simulink library "dyn"  (Simulink 8.2)
settings: Solver=ode45  StartTime=0.0  StopTime=10.0  RelTol=1e-3
undefined symbols (not defined in the file or in its folder): KVSE_AccelWeightOffset_rat, KVSE_AccelWeightSlope_rat, KVSE_StartModeInDelaySpd_kph, KVSE_StartModeInWheelSpd_kph, KVSE_StartModeOutWheelSpd_kph, KVSE_TurnModeInYawRate_degps, KVSE_TurnModeOutYawRate_degps, KVSE_WheelSpdAdjust_rat, KVSE_WheelWeightOffset_rat, KVSE_WheelWeightSlope_rat
libraries: simulink x6
(part 1 of 2)
settings Model: RequirementInfo="{}  %GIDa_9c3e9883_6bb3_4e31_949e_ba791919a9a8"  Creator=16027  LastModifiedBy=14014  CovModelRefEnable=off

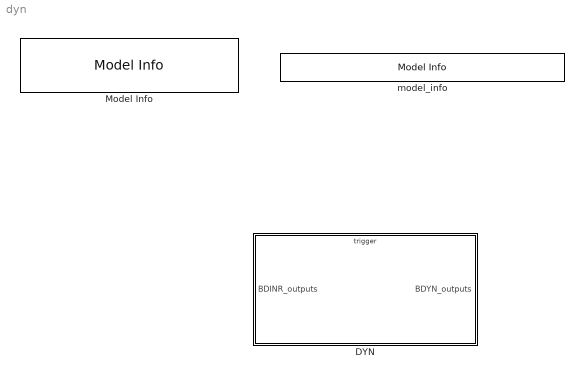
== system dyn ==
  DYN : Subsystem
  Model Info : simulink/Model-Wide Utilities/Model Info  InitialBlockCM=None  BlockCM=none  Frame=on  DisplayStringWithTags=|  HorizontalTextAlignment=Left  LeftAlignmentValue=0.02  SourceBlockDiagram=dyn  TagMaxNumber=20
      | Model Version        : %<ModelVersion>
      | Creator                   : %<Creator>
      | Last Modified by    : %<LastModifiedBy>
  model_info : simulink/Model-Wide Utilities/Model Info  InitialBlockCM=None  BlockCM=None  Frame=on  DisplayStringWithTags=$Id: dyn.mdl 1524 2016-11-04 02:29:39Z chimotsai $  HorizontalTextAlignment=Center  LeftAlignmentValue=0.5  SourceBlockDiagram=dyn  TagMaxNumber=20

== system dyn/DYN ==
  BDINR_outputs : Inport  OutDataTypeStr=Bus: BDINR_outputs
  trig_DYN : TriggerPort  TriggerType=function-call  PortDimensions=1
  Bus Creator : BusCreator  Inputs=1  OutDataTypeStr=Bus: BDYN_outputs
  Bus Selector1 : BusSelector  OutputSignals=VDINR_RRWheelSpeed_kph,VDINR_LRWheelSpeed_kph,VDINR_RFWheelSpeed_kph,VDINR_LFWheelSpeed_kph,VDINR_LongAccel_G,VDINR_YawRate_degps
  Vehicle Speed Estimation : Subsystem  RequirementInfo={} %GIDa_6aef2b2b_4aef_4102_9e64_605181178381
  BDYN_outputs : Outport  OutDataTypeStr=Bus: BDYN_outputs
  wires:
  Bus Selector1/1 -> Vehicle Speed Estimation/1(VDINR_RRWheelSpeed_kph)  "<VDINR_RRWheelSpeed_kph>"
  Vehicle Speed Estimation/1(VVSE_VehSpdEst_kph) -> Bus Creator/1
  BDINR_outputs/1 -> Bus Selector1/1
  Bus Creator/1 -> BDYN_outputs/1  "BDYN_outputs"
  Bus Selector1/2 -> Vehicle Speed Estimation/2(VDINR_LRWheelSpeed_kph)  "<VDINR_LRWheelSpeed_kph>"
  Bus Selector1/3 -> Vehicle Speed Estimation/3(VDINR_RFWheelSpeed_kph)  "<VDINR_RFWheelSpeed_kph>"
  Bus Selector1/4 -> Vehicle Speed Estimation/4(VDINR_LFWheelSpeed_kph)  "<VDINR_LFWheelSpeed_kph>"
  Bus Selector1/5 -> Vehicle Speed Estimation/5(VDINR_LongAccel_G)  "<VDINR_LongAccel_G>"
  Bus Selector1/6 -> Vehicle Speed Estimation/6(VDINR_YawRate_degps)  "<VDINR_YawRate_degps>"

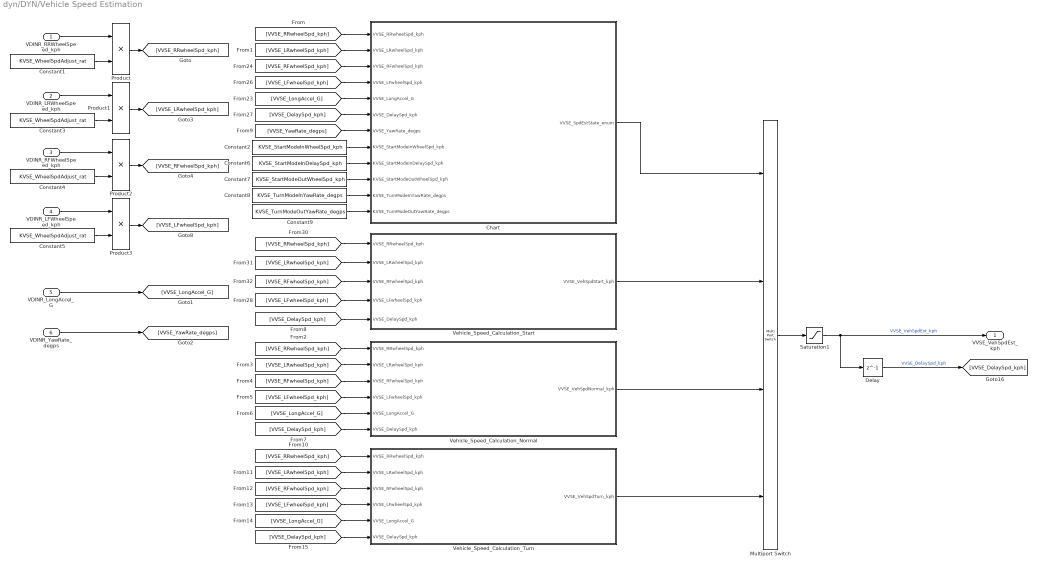
== system dyn/DYN/Vehicle Speed Estimation ==
  VDINR_RRWheelSpeed_kph : Inport
  VDINR_LRWheelSpeed_kph : Inport  Port=2
  VDINR_RFWheelSpeed_kph : Inport  Port=3
  VDINR_LFWheelSpeed_kph : Inport  Port=4
  VDINR_LongAccel_G : Inport  Port=5
  VDINR_YawRate_degps : Inport  Port=6
  Chart : Stateflow chart  TreatAsAtomicUnit=on
  Constant{1,3..5} (4 alike) : Constant  Value=KVSE_WheelSpdAdjust_rat
  Constant2 : Constant  Value=KVSE_StartModeInWheelSpd_kph
  Constant6 : Constant  Value=KVSE_StartModeInDelaySpd_kph
  Constant7 : Constant  Value=KVSE_StartModeOutWheelSpd_kph
  Constant8 : Constant  Value=KVSE_TurnModeInYawRate_degps
  Constant9 : Constant  Value=KVSE_TurnModeOutYawRate_degps
  Delay : Delay  DelayLength=1  InitialCondition=0
  Multiport Switch : MultiPortSwitch
  Product{,1..3} (4 alike) : Product
  Saturation1 : Saturate  UpperLimit=220  LowerLimit=0
  "Vehicle_Speed_Calculation_Normal " : Subsystem
  Vehicle_Speed_Calculation_Start : Subsystem
  "Vehicle_Speed_Calculation_Turn " : Subsystem
  VVSE_VehSpdEst_kph : Outport
  wires:
  Delay/1 -> [VVSE_DelaySpd_kph]  "VVSE_DelaySpd_kph"
  Saturation1/1 -> VVSE_VehSpdEst_kph/1, Delay/1  "VVSE_VehSpdEst_kph"
  [VVSE_LRwheelSpd_kph] -> "Vehicle_Speed_Calculation_Normal "/2(VVSE_LRwheelSpd_kph)
  [VVSE_RFwheelSpd_kph] -> "Vehicle_Speed_Calculation_Normal "/3(VVSE_RFwheelSpd_kph)
  [VVSE_LFwheelSpd_kph] -> "Vehicle_Speed_Calculation_Normal "/4(VVSE_LFwheelSpd_kph)
  [VVSE_LongAccel_G] -> "Vehicle_Speed_Calculation_Normal "/5(VVSE_LongAccel_G)
  [VVSE_DelaySpd_kph] -> "Vehicle_Speed_Calculation_Normal "/6(VVSE_DelaySpd_kph)
  [VVSE_RRwheelSpd_kph] -> Chart/1(VVSE_RRwheelSpd_kph)
  [VVSE_LRwheelSpd_kph] -> Chart/2(VVSE_LRwheelSpd_kph)
  [VVSE_LFwheelSpd_kph] -> Chart/4(VVSE_LFwheelSpd_kph)
  [VVSE_RFwheelSpd_kph] -> Chart/3(VVSE_RFwheelSpd_kph)
  [VVSE_DelaySpd_kph] -> Chart/6(VVSE_DelaySpd_kph)
  [VVSE_LongAccel_G] -> Chart/5(VVSE_LongAccel_G)
  Multiport Switch/1 -> Saturation1/1
  [VVSE_RRwheelSpd_kph] -> "Vehicle_Speed_Calculation_Normal "/1(VVSE_RRwheelSpd_kph)
  [VVSE_LFwheelSpd_kph] -> Vehicle_Speed_Calculation_Start/4(VVSE_LFwheelSpd_kph)
  [VVSE_RFwheelSpd_kph] -> Vehicle_Speed_Calculation_Start/3(VVSE_RFwheelSpd_kph)
  [VVSE_LRwheelSpd_kph] -> Vehicle_Speed_Calculation_Start/2(VVSE_LRwheelSpd_kph)
  [VVSE_RRwheelSpd_kph] -> Vehicle_Speed_Calculation_Start/1(VVSE_RRwheelSpd_kph)
  [VVSE_DelaySpd_kph] -> Vehicle_Speed_Calculation_Start/5(VVSE_DelaySpd_kph)
  Product/1 -> [VVSE_RRwheelSpd_kph]
  VDINR_RRWheelSpeed_kph/1 -> Product/1
  Constant1/1 -> Product/2
  Product1/1 -> [VVSE_LRwheelSpd_kph]
  VDINR_LRWheelSpeed_kph/1 -> Product1/1
  Constant3/1 -> Product1/2
  Product2/1 -> [VVSE_RFwheelSpd_kph]
  VDINR_RFWheelSpeed_kph/1 -> Product2/1
  Constant4/1 -> Product2/2
  Product3/1 -> [VVSE_LFwheelSpd_kph]
  VDINR_LFWheelSpeed_kph/1 -> Product3/1
  Constant5/1 -> Product3/2
  VDINR_LongAccel_G/1 -> [VVSE_LongAccel_G]
  "Vehicle_Speed_Calculation_Normal "/1(VVSE_VehSpdNormal_kph) -> Multiport Switch/3
  Vehicle_Speed_Calculation_Start/1(VVSE_VehSpdStart_kph) -> Multiport Switch/2
  VDINR_YawRate_degps/1 -> [VVSE_YawRate_degps]
  [VVSE_YawRate_degps] -> Chart/7(VVSE_YawRate_degps)
  Chart/1(VVSE_SpdEstState_enum) -> Multiport Switch/1
  "Vehicle_Speed_Calculation_Turn "/1(VVSE_VehSpdTurn_kph) -> Multiport Switch/4
  [VVSE_RRwheelSpd_kph] -> "Vehicle_Speed_Calculation_Turn "/1(VVSE_RRwheelSpd_kph)
  [VVSE_LRwheelSpd_kph] -> "Vehicle_Speed_Calculation_Turn "/2(VVSE_LRwheelSpd_kph)
  [VVSE_RFwheelSpd_kph] -> "Vehicle_Speed_Calculation_Turn "/3(VVSE_RFwheelSpd_kph)
  [VVSE_LFwheelSpd_kph] -> "Vehicle_Speed_Calculation_Turn "/4(VVSE_LFwheelSpd_kph)
  [VVSE_LongAccel_G] -> "Vehicle_Speed_Calculation_Turn "/5(VVSE_LongAccel_G)
  [VVSE_DelaySpd_kph] -> "Vehicle_Speed_Calculation_Turn "/6(VVSE_DelaySpd_kph)
  Constant2/1 -> Chart/8(KVSE_StartModeInWheelSpd_kph)
  Constant6/1 -> Chart/9(KVSE_StartModeInDelaySpd_kph)
  Constant7/1 -> Chart/10(KVSE_StartModeOutWheelSpd_kph)
  Constant8/1 -> Chart/11(KVSE_TurnModeInYawRate_degps)
  Constant9/1 -> Chart/12(KVSE_TurnModeOutYawRate_degps)

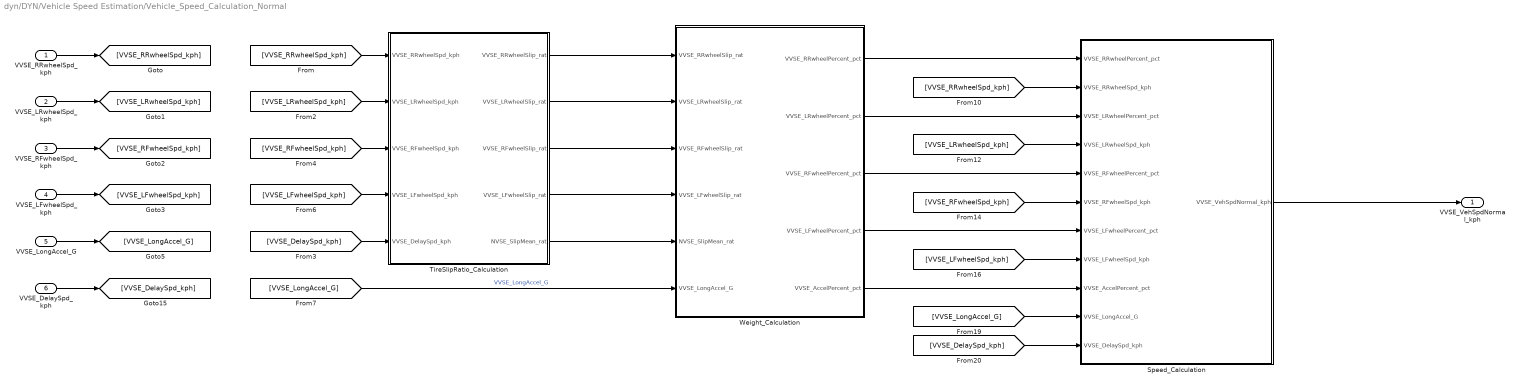
== system dyn/DYN/Vehicle Speed Estimation/Vehicle_Speed_Calculation_Normal  ==
  VVSE_RRwheelSpd_kph : Inport
  VVSE_LRwheelSpd_kph : Inport  Port=2
  VVSE_RFwheelSpd_kph : Inport  Port=3
  VVSE_LFwheelSpd_kph : Inport  Port=4
  VVSE_LongAccel_G : Inport  Port=5
  VVSE_DelaySpd_kph : Inport  Port=6
  Speed_Calculation : Subsystem
  TireSlipRatio_Calculation : Subsystem
  Weight_Calculation : Subsystem  RequirementInfo={} %GIDa_581bf922_3c60_4f28_b9a5_a6cc319ffbb8
  VVSE_VehSpdNormal_kph : Outport
  wires:
  [VVSE_RRwheelSpd_kph] -> TireSlipRatio_Calculation/1(VVSE_RRwheelSpd_kph)
  [VVSE_LongAccel_G] -> Weight_Calculation/6(VVSE_LongAccel_G)  "VVSE_LongAccel_G"
  Speed_Calculation/1(VVSE_VehSpdNormal_kph) -> VVSE_VehSpdNormal_kph/1
  VVSE_LongAccel_G/1 -> [VVSE_LongAccel_G]
  VVSE_DelaySpd_kph/1 -> [VVSE_DelaySpd_kph]
  Weight_Calculation/5(VVSE_AccelPercent_pct) -> Speed_Calculation/9(VVSE_AccelPercent_pct)
  [VVSE_LongAccel_G] -> Speed_Calculation/10(VVSE_LongAccel_G)
  [VVSE_DelaySpd_kph] -> Speed_Calculation/11(VVSE_DelaySpd_kph)
  Weight_Calculation/2(VVSE_LRwheelPercent_pct) -> Speed_Calculation/3(VVSE_LRwheelPercent_pct)
  [VVSE_RRwheelSpd_kph] -> Speed_Calculation/2(VVSE_RRwheelSpd_kph)
  Weight_Calculation/1(VVSE_RRwheelPercent_pct) -> Speed_Calculation/1(VVSE_RRwheelPercent_pct)
  [VVSE_LRwheelSpd_kph] -> Speed_Calculation/4(VVSE_LRwheelSpd_kph)
  Weight_Calculation/3(VVSE_RFwheelPercent_pct) -> Speed_Calculation/5(VVSE_RFwheelPercent_pct)
  [VVSE_RFwheelSpd_kph] -> Speed_Calculation/6(VVSE_RFwheelSpd_kph)
  Weight_Calculation/4(VVSE_LFwheelPercent_pct) -> Speed_Calculation/7(VVSE_LFwheelPercent_pct)
  VVSE_LRwheelSpd_kph/1 -> [VVSE_LRwheelSpd_kph]
  VVSE_RFwheelSpd_kph/1 -> [VVSE_RFwheelSpd_kph]
  VVSE_LFwheelSpd_kph/1 -> [VVSE_LFwheelSpd_kph]
  VVSE_RRwheelSpd_kph/1 -> [VVSE_RRwheelSpd_kph]
  [VVSE_LRwheelSpd_kph] -> TireSlipRatio_Calculation/2(VVSE_LRwheelSpd_kph)
  [VVSE_RFwheelSpd_kph] -> TireSlipRatio_Calculation/3(VVSE_RFwheelSpd_kph)
  [VVSE_LFwheelSpd_kph] -> TireSlipRatio_Calculation/4(VVSE_LFwheelSpd_kph)
  [VVSE_DelaySpd_kph] -> TireSlipRatio_Calculation/5(VVSE_DelaySpd_kph)
  TireSlipRatio_Calculation/5(NVSE_SlipMean_rat) -> Weight_Calculation/5(NVSE_SlipMean_rat)
  TireSlipRatio_Calculation/4(VVSE_LFwheelSlip_rat) -> Weight_Calculation/4(VVSE_LFwheelSlip_rat)
  TireSlipRatio_Calculation/3(VVSE_RFwheelSlip_rat) -> Weight_Calculation/3(VVSE_RFwheelSlip_rat)
  TireSlipRatio_Calculation/2(VVSE_LRwheelSlip_rat) -> Weight_Calculation/2(VVSE_LRwheelSlip_rat)
  TireSlipRatio_Calculation/1(VVSE_RRwheelSlip_rat) -> Weight_Calculation/1(VVSE_RRwheelSlip_rat)
  [VVSE_LFwheelSpd_kph] -> Speed_Calculation/8(VVSE_LFwheelSpd_kph)

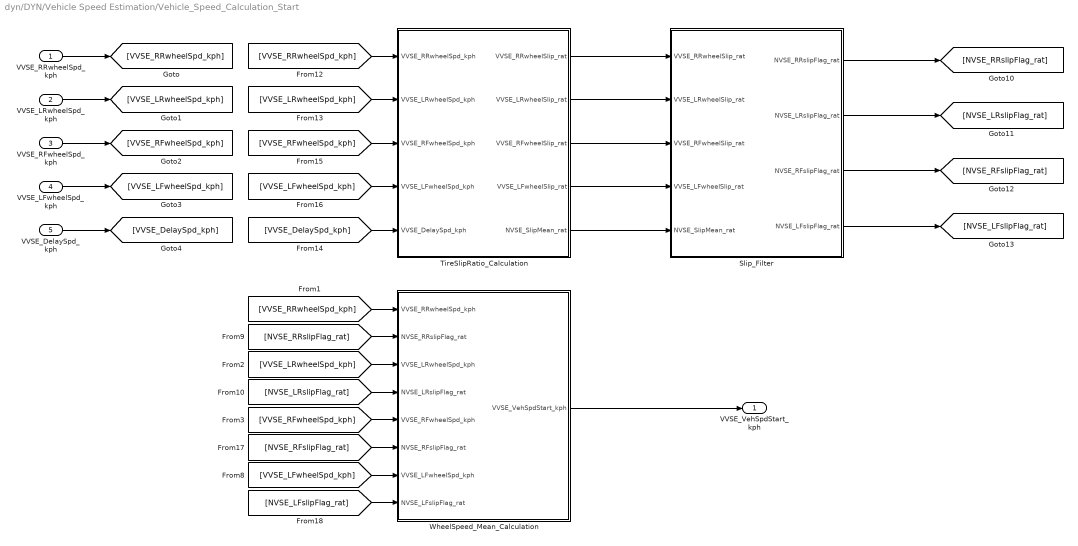
== system dyn/DYN/Vehicle Speed Estimation/Vehicle_Speed_Calculation_Start ==
  VVSE_RRwheelSpd_kph : Inport
  VVSE_LRwheelSpd_kph : Inport  Port=2
  VVSE_RFwheelSpd_kph : Inport  Port=3
  VVSE_LFwheelSpd_kph : Inport  Port=4
  VVSE_DelaySpd_kph : Inport  Port=5
  Slip_Filter : Subsystem
  TireSlipRatio_Calculation : Subsystem  RequirementInfo={} %GIDa_4f43d894_ac8b_41fb_96be_b9fe366c055a
  WheelSpeed_Mean_Calculation : Subsystem
  VVSE_VehSpdStart_kph : Outport
  wires:
  VVSE_LRwheelSpd_kph/1 -> [VVSE_LRwheelSpd_kph]
  VVSE_RFwheelSpd_kph/1 -> [VVSE_RFwheelSpd_kph]
  VVSE_LFwheelSpd_kph/1 -> [VVSE_LFwheelSpd_kph]
  VVSE_RRwheelSpd_kph/1 -> [VVSE_RRwheelSpd_kph]
  [VVSE_RRwheelSpd_kph] -> TireSlipRatio_Calculation/1(VVSE_RRwheelSpd_kph)
  [VVSE_LRwheelSpd_kph] -> TireSlipRatio_Calculation/2(VVSE_LRwheelSpd_kph)
  [VVSE_DelaySpd_kph] -> TireSlipRatio_Calculation/5(VVSE_DelaySpd_kph)
  [VVSE_LFwheelSpd_kph] -> TireSlipRatio_Calculation/4(VVSE_LFwheelSpd_kph)
  [VVSE_RFwheelSpd_kph] -> TireSlipRatio_Calculation/3(VVSE_RFwheelSpd_kph)
  VVSE_DelaySpd_kph/1 -> [VVSE_DelaySpd_kph]
  Slip_Filter/1(NVSE_RRslipFlag_rat) -> [NVSE_RRslipFlag_rat]
  Slip_Filter/2(NVSE_LRslipFlag_rat) -> [NVSE_LRslipFlag_rat]
  Slip_Filter/3(NVSE_RFslipFlag_rat) -> [NVSE_RFslipFlag_rat]
  Slip_Filter/4(NVSE_LFslipFlag_rat) -> [NVSE_LFslipFlag_rat]
  [VVSE_RRwheelSpd_kph] -> WheelSpeed_Mean_Calculation/1(VVSE_RRwheelSpd_kph)
  [NVSE_RRslipFlag_rat] -> WheelSpeed_Mean_Calculation/2(NVSE_RRslipFlag_rat)
  [VVSE_LRwheelSpd_kph] -> WheelSpeed_Mean_Calculation/3(VVSE_LRwheelSpd_kph)
  [NVSE_LRslipFlag_rat] -> WheelSpeed_Mean_Calculation/4(NVSE_LRslipFlag_rat)
  [VVSE_RFwheelSpd_kph] -> WheelSpeed_Mean_Calculation/5(VVSE_RFwheelSpd_kph)
  [NVSE_RFslipFlag_rat] -> WheelSpeed_Mean_Calculation/6(NVSE_RFslipFlag_rat)
  [VVSE_LFwheelSpd_kph] -> WheelSpeed_Mean_Calculation/7(VVSE_LFwheelSpd_kph)
  [NVSE_LFslipFlag_rat] -> WheelSpeed_Mean_Calculation/8(NVSE_LFslipFlag_rat)
  WheelSpeed_Mean_Calculation/1(VVSE_VehSpdStart_kph) -> VVSE_VehSpdStart_kph/1
  TireSlipRatio_Calculation/1(VVSE_RRwheelSlip_rat) -> Slip_Filter/1(VVSE_RRwheelSlip_rat)
  TireSlipRatio_Calculation/2(VVSE_LRwheelSlip_rat) -> Slip_Filter/2(VVSE_LRwheelSlip_rat)
  TireSlipRatio_Calculation/3(VVSE_RFwheelSlip_rat) -> Slip_Filter/3(VVSE_RFwheelSlip_rat)
  TireSlipRatio_Calculation/4(VVSE_LFwheelSlip_rat) -> Slip_Filter/4(VVSE_LFwheelSlip_rat)
  TireSlipRatio_Calculation/5(NVSE_SlipMean_rat) -> Slip_Filter/5(NVSE_SlipMean_rat)

== system dyn/DYN/Vehicle Speed Estimation/Vehicle_Speed_Calculation_Turn  ==
  VVSE_RRwheelSpd_kph : Inport
  VVSE_LRwheelSpd_kph : Inport  Port=2
  VVSE_RFwheelSpd_kph : Inport  Port=3
  VVSE_LFwheelSpd_kph : Inport  Port=4
  VVSE_LongAccel_G : Inport  Port=5
  VVSE_DelaySpd_kph : Inport  Port=6
  Speed_Calculation1 : Subsystem
  TireSlipRatio_Calculation1 : Subsystem  AncestorBlock=VSE/VSE/Vehicle Speed Estimation/Vehicle_Speed_Calculation_Normal /TireSlipRatio_Calculation
  Weight_Calculation : Subsystem
  VVSE_VehSpdTurn_kph : Outport
  wires:
  [VVSE_RRwheelSpd_kph] -> TireSlipRatio_Calculation1/1(VVSE_RRwheelSpd_kph)
  [VVSE_LongAccel_G] -> Weight_Calculation/6(VVSE_LongAccel_G)  "VVSE_LongAccel_G"
  Speed_Calculation1/1(VVSE_VehSpdTurn_kph) -> VVSE_VehSpdTurn_kph/1
  VVSE_LongAccel_G/1 -> [VVSE_LongAccel_G]
  VVSE_DelaySpd_kph/1 -> [VVSE_DelaySpd_kph]
  Weight_Calculation/5(VVSE_AccelPercent_pct) -> Speed_Calculation1/9(VVSE_AccelPercent_pct)
  [VVSE_LongAccel_G] -> Speed_Calculation1/10(VVSE_LongAccel_G)
  [VVSE_DelaySpd_kph] -> Speed_Calculation1/11(VVSE_DelaySpd_kph)
  Weight_Calculation/2(VVSE_LRwheelPercent_pct) -> Speed_Calculation1/3(VVSE_LRwheelPercent_pct)
  [VVSE_RRwheelSpd_kph] -> Speed_Calculation1/2(VVSE_RRwheelSpd_kph)
  Weight_Calculation/1(VVSE_RRwheelPercent_pct) -> Speed_Calculation1/1(VVSE_RRwheelPercent_pct)
  [VVSE_LRwheelSpd_kph] -> Speed_Calculation1/4(VVSE_LRwheelSpd_kph)
  Weight_Calculation/3(VVSE_RFwheelPercent_pct) -> Speed_Calculation1/5(VVSE_RFwheelPercent_pct)
  [VVSE_RFwheelSpd_kph] -> Speed_Calculation1/6(VVSE_RFwheelSpd_kph)
  Weight_Calculation/4(VVSE_LFwheelPercent_pct) -> Speed_Calculation1/7(VVSE_LFwheelPercent_pct)
  VVSE_LRwheelSpd_kph/1 -> [VVSE_LRwheelSpd_kph]
  VVSE_RFwheelSpd_kph/1 -> [VVSE_RFwheelSpd_kph]
  VVSE_LFwheelSpd_kph/1 -> [VVSE_LFwheelSpd_kph]
  VVSE_RRwheelSpd_kph/1 -> [VVSE_RRwheelSpd_kph]
  [VVSE_LRwheelSpd_kph] -> TireSlipRatio_Calculation1/2(VVSE_LRwheelSpd_kph)
  [VVSE_RFwheelSpd_kph] -> TireSlipRatio_Calculation1/3(VVSE_RFwheelSpd_kph)
  [VVSE_LFwheelSpd_kph] -> TireSlipRatio_Calculation1/4(VVSE_LFwheelSpd_kph)
  TireSlipRatio_Calculation1/5(NVSE_SlipMean_rat) -> Weight_Calculation/5(NVSE_SlipMean_rat)
  TireSlipRatio_Calculation1/4(VVSE_LFwheelSlip_rat) -> Weight_Calculation/4(VVSE_LFwheelSlip_rat)
  TireSlipRatio_Calculation1/3(VVSE_RFwheelSlip_rat) -> Weight_Calculation/3(VVSE_RFwheelSlip_rat)
  TireSlipRatio_Calculation1/2(VVSE_LRwheelSlip_rat) -> Weight_Calculation/2(VVSE_LRwheelSlip_rat)
  TireSlipRatio_Calculation1/1(VVSE_RRwheelSlip_rat) -> Weight_Calculation/1(VVSE_RRwheelSlip_rat)
  [VVSE_LFwheelSpd_kph] -> Speed_Calculation1/8(VVSE_LFwheelSpd_kph)

== system dyn/DYN/Vehicle Speed Estimation/Vehicle_Speed_Calculation_Normal /Speed_Calculation ==
  VVSE_RRwheelPercent_pct : Inport
  VVSE_RRwheelSpd_kph : Inport  Port=2
  VVSE_LRwheelPercent_pct : Inport  Port=3
  VVSE_LRwheelSpd_kph : Inport  Port=4
  VVSE_RFwheelPercent_pct : Inport  Port=5
  VVSE_RFwheelSpd_kph : Inport  Port=6
  VVSE_LFwheelPercent_pct : Inport  Port=7
  VVSE_LFwheelSpd_kph : Inport  Port=8
  VVSE_AccelPercent_pct : Inport  Port=9
  VVSE_LongAccel_G : Inport  Port=10
  VVSE_DelaySpd_kph : Inport  Port=11
  Add : Sum
  Add1 : Sum  Inputs=+++++
  Gain : Gain  Gain=9.81
  Gain1 : Gain  Gain=0.01
  Gain2 : Gain  Gain=3.6
  Product{,1..4} (5 alike) : Product
  VVSE_VehSpdNormal_kph : Outport
  wires:
  Gain/1 -> Gain1/1
  Product4/1 -> Add1/5
  Product/1 -> Add1/1
  Add/1 -> Product4/2
  Product1/1 -> Add1/2
  Product2/1 -> Add1/3
  Gain2/1 -> Add/1
  Product3/1 -> Add1/4
  Gain1/1 -> Gain2/1
  VVSE_RRwheelPercent_pct/1 -> Product/1
  VVSE_RFwheelPercent_pct/1 -> Product2/1
  VVSE_LongAccel_G/1 -> Gain/1
  VVSE_DelaySpd_kph/1 -> Add/2
  VVSE_LRwheelPercent_pct/1 -> Product1/1
  VVSE_LRwheelSpd_kph/1 -> Product1/2
  VVSE_AccelPercent_pct/1 -> Product4/1
  VVSE_LFwheelSpd_kph/1 -> Product3/2
  VVSE_RRwheelSpd_kph/1 -> Product/2
  VVSE_RFwheelSpd_kph/1 -> Product2/2
  VVSE_LFwheelPercent_pct/1 -> Product3/1
  Add1/1 -> VVSE_VehSpdNormal_kph/1  "VVSE_VehSpdNormal_kph"

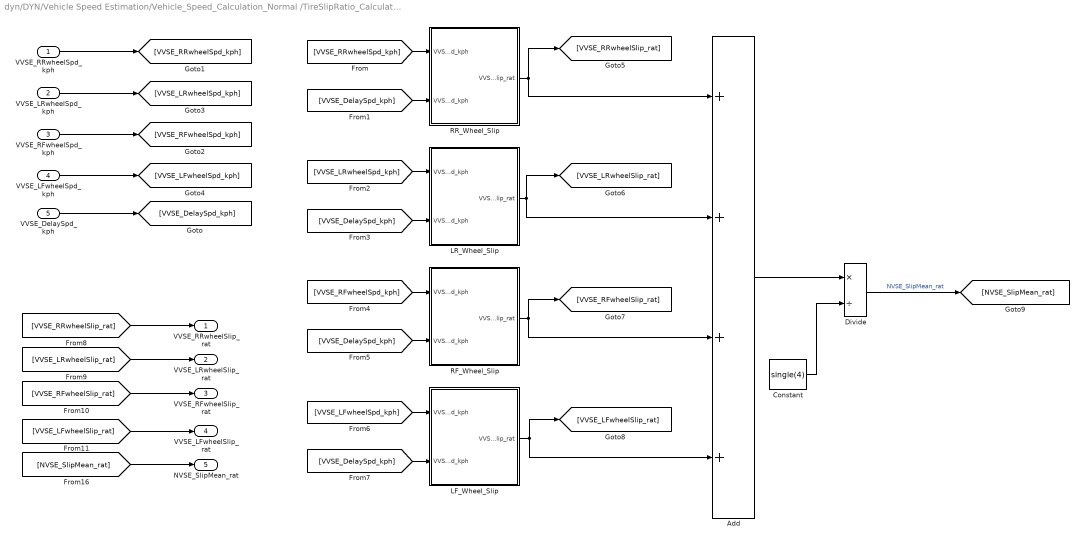
== system dyn/DYN/Vehicle Speed Estimation/Vehicle_Speed_Calculation_Normal /TireSlipRatio_Calculation ==
  VVSE_RRwheelSpd_kph : Inport
  VVSE_LRwheelSpd_kph : Inport  Port=2
  VVSE_RFwheelSpd_kph : Inport  Port=3
  VVSE_LFwheelSpd_kph : Inport  Port=4
  VVSE_DelaySpd_kph : Inport  Port=5
  Add : Sum  Inputs=++++
  Constant : Constant  Value=single(4)
  Divide : Product  Inputs=*/
  "LF_Wheel_Slip " : Subsystem
  LR_Wheel_Slip : Subsystem
  RF_Wheel_Slip : Subsystem
  RR_Wheel_Slip : Subsystem  RequirementInfo={} %GIDa_c8b2f6a2_3d64_4d29_9794_b0dc0d6a5f58
  VVSE_RRwheelSlip_rat : Outport
  VVSE_LRwheelSlip_rat : Outport  Port=2
  VVSE_RFwheelSlip_rat : Outport  Port=3
  VVSE_LFwheelSlip_rat : Outport  Port=4
  NVSE_SlipMean_rat : Outport  Port=5
  wires:
  Constant/1 -> Divide/2
  VVSE_DelaySpd_kph/1 -> [VVSE_DelaySpd_kph]
  Divide/1 -> [NVSE_SlipMean_rat]  "NVSE_SlipMean_rat"
  Add/1 -> Divide/1
  "LF_Wheel_Slip "/1(VVSE_LFwheelSlip_rat) -> [VVSE_LFwheelSlip_rat], Add/4
  [NVSE_SlipMean_rat] -> NVSE_SlipMean_rat/1
  [VVSE_DelaySpd_kph] -> RR_Wheel_Slip/2(VVSE_DelaySpd_kph)
  [VVSE_LRwheelSlip_rat] -> VVSE_LRwheelSlip_rat/1
  [VVSE_LFwheelSlip_rat] -> VVSE_LFwheelSlip_rat/1
  VVSE_RRwheelSpd_kph/1 -> [VVSE_RRwheelSpd_kph]
  RF_Wheel_Slip/1(VVSE_RFwheelSlip_rat) -> [VVSE_RFwheelSlip_rat], Add/3
  RR_Wheel_Slip/1(VVSE_RRwheelSlip_rat) -> [VVSE_RRwheelSlip_rat], Add/1
  [VVSE_RRwheelSlip_rat] -> VVSE_RRwheelSlip_rat/1
  [VVSE_RFwheelSlip_rat] -> VVSE_RFwheelSlip_rat/1
  VVSE_RFwheelSpd_kph/1 -> [VVSE_RFwheelSpd_kph]
  LR_Wheel_Slip/1(VVSE_LRwheelSlip_rat) -> Add/2, [VVSE_LRwheelSlip_rat]
  [VVSE_RFwheelSpd_kph] -> RF_Wheel_Slip/1(VVSE_RFwheelSpd_kph)
  [VVSE_DelaySpd_kph] -> RF_Wheel_Slip/2(VVSE_DelaySpd_kph)
  [VVSE_LRwheelSpd_kph] -> LR_Wheel_Slip/1(VVSE_LRwheelSpd_kph)
  VVSE_LFwheelSpd_kph/1 -> [VVSE_LFwheelSpd_kph]
  VVSE_LRwheelSpd_kph/1 -> [VVSE_LRwheelSpd_kph]
  [VVSE_DelaySpd_kph] -> LR_Wheel_Slip/2(VVSE_DelaySpd_kph)
  [VVSE_DelaySpd_kph] -> "LF_Wheel_Slip "/2(VVSE_DelaySpd_kph)
  [VVSE_LFwheelSpd_kph] -> "LF_Wheel_Slip "/1(VVSE_LFwheelSpd_kph)
  [VVSE_RRwheelSpd_kph] -> RR_Wheel_Slip/1(VVSE_RRwheelSpd_kph)

== system dyn/DYN/Vehicle Speed Estimation/Vehicle_Speed_Calculation_Normal /Weight_Calculation ==
  VVSE_RRwheelSlip_rat : Inport
  VVSE_LRwheelSlip_rat : Inport  Port=2
  VVSE_RFwheelSlip_rat : Inport  Port=3
  VVSE_LFwheelSlip_rat : Inport  Port=4
  NVSE_SlipMean_rat : Inport  Port=5
  VVSE_LongAccel_G : Inport  Port=6
  Percentage : Subsystem  RequirementInfo={} %GIDa_b7f10889_7b75_40d3_8cb6_4d2c6f0c621d
  Weight : Subsystem  RequirementInfo={} %GIDa_ee7ecb5e_3ba9_4a62_b515_b78ff1211ee4
  VVSE_RRwheelPercent_pct : Outport
  VVSE_LRwheelPercent_pct : Outport  Port=2
  VVSE_RFwheelPercent_pct : Outport  Port=3
  VVSE_LFwheelPercent_pct : Outport  Port=4
  VVSE_AccelPercent_pct : Outport  Port=5
  wires:
  Percentage/1(VVSE_RRwheelPercent_pct) -> VVSE_RRwheelPercent_pct/1
  Percentage/2(VVSE_LRwheelPercent_pct) -> VVSE_LRwheelPercent_pct/1
  Percentage/3(VVSE_RFwheelPercent_pct) -> VVSE_RFwheelPercent_pct/1
  Percentage/4(VVSE_LFwheelPercent_pct) -> VVSE_LFwheelPercent_pct/1
  Percentage/5(VVSE_AccelPercent_pct) -> VVSE_AccelPercent_pct/1
  VVSE_RRwheelSlip_rat/1 -> Weight/1(VVSE_RRwheelSlip_rat)
  VVSE_LRwheelSlip_rat/1 -> Weight/2(VVSE_LRwheelSlip_rat)
  VVSE_RFwheelSlip_rat/1 -> Weight/3(VVSE_RFwheelSlip_rat)
  VVSE_LFwheelSlip_rat/1 -> Weight/4(VVSE_LFwheelSlip_rat)
  VVSE_LongAccel_G/1 -> Weight/6(VVSE_LongAccel_G)
  Weight/1(NVSE_RRwheelWeight_rat) -> Percentage/1(NVSE_RRwheelWeight_rat)
  Weight/2(NVSE_LRwheelWeight_rat) -> Percentage/2(NVSE_LRwheelWeight_rat)
  Weight/3(NVSE_RFwheelWeight_rat) -> Percentage/3(NVSE_RFwheelWeight_rat)
  Weight/4(NVSE_LFwheelWeight_rat) -> Percentage/4(NVSE_LFwheelWeight_rat)
  Weight/5(NVSE_AccelWeight_rat) -> Percentage/5(NVSE_AccelWeight_rat)
  NVSE_SlipMean_rat/1 -> Weight/5(NVSE_SlipMean_rat)

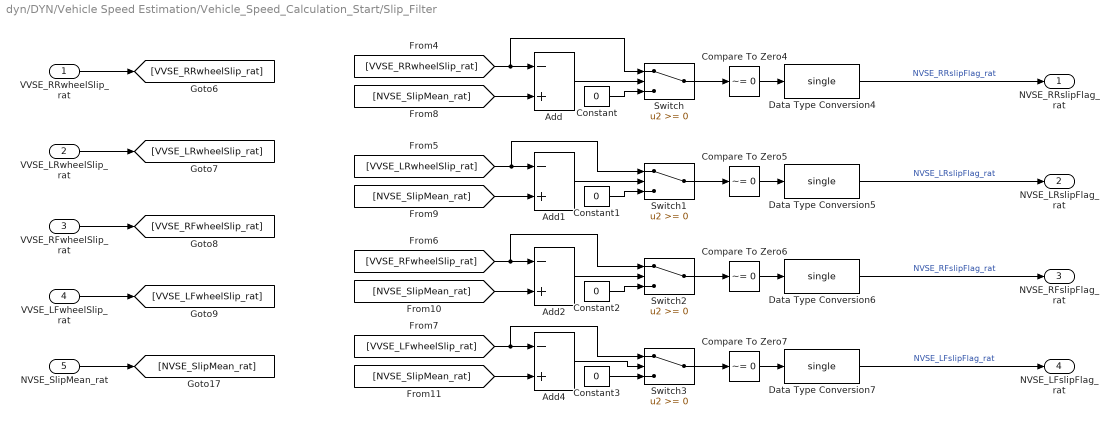
== system dyn/DYN/Vehicle Speed Estimation/Vehicle_Speed_Calculation_Start/Slip_Filter ==
  VVSE_RRwheelSlip_rat : Inport
  VVSE_LRwheelSlip_rat : Inport  Port=2
  VVSE_RFwheelSlip_rat : Inport  Port=3
  VVSE_LFwheelSlip_rat : Inport  Port=4
  NVSE_SlipMean_rat : Inport  Port=5
  Add{,1..2,4} (4 alike) : Sum  Inputs=-+
  Compare To Zero{4..7} (4 alike) : simulink/Logic and Bit Operations/Compare To Zero  relop=~=  OutDataTypeStr=boolean
  Constant{,1..3} (4 alike) : Constant  Value=0
  Data Type Conversion{4..7} (4 alike) : DataTypeConversion  OutDataTypeStr=single
  Switch{,1..3} (4 alike) : Switch
  NVSE_RRslipFlag_rat : Outport
  NVSE_LRslipFlag_rat : Outport  Port=2
  NVSE_RFslipFlag_rat : Outport  Port=3
  NVSE_LFslipFlag_rat : Outport  Port=4
  wires:
  Constant/1 -> Switch/3
  Add/1 -> Switch/2
  Compare To Zero7/1 -> Data Type Conversion7/1
  Compare To Zero6/1 -> Data Type Conversion6/1
  Compare To Zero5/1 -> Data Type Conversion5/1
  Constant1/1 -> Switch1/3
  Add1/1 -> Switch1/2
  Constant2/1 -> Switch2/3
  Add2/1 -> Switch2/2
  Constant3/1 -> Switch3/3
  Add4/1 -> Switch3/2
  [VVSE_RRwheelSlip_rat] -> Add/1, Switch/1
  [NVSE_SlipMean_rat] -> Add/2
  [VVSE_LRwheelSlip_rat] -> Add1/1, Switch1/1
  [NVSE_SlipMean_rat] -> Add1/2
  [NVSE_SlipMean_rat] -> Add2/2
  [VVSE_RFwheelSlip_rat] -> Add2/1, Switch2/1
  [NVSE_SlipMean_rat] -> Add4/2
  [VVSE_LFwheelSlip_rat] -> Add4/1, Switch3/1
  VVSE_RRwheelSlip_rat/1 -> [VVSE_RRwheelSlip_rat]
  VVSE_LRwheelSlip_rat/1 -> [VVSE_LRwheelSlip_rat]
  VVSE_RFwheelSlip_rat/1 -> [VVSE_RFwheelSlip_rat]
  VVSE_LFwheelSlip_rat/1 -> [VVSE_LFwheelSlip_rat]
  NVSE_SlipMean_rat/1 -> [NVSE_SlipMean_rat]
  Switch/1 -> Compare To Zero4/1
  Compare To Zero4/1 -> Data Type Conversion4/1
  Switch1/1 -> Compare To Zero5/1
  Switch2/1 -> Compare To Zero6/1
  Switch3/1 -> Compare To Zero7/1
  Data Type Conversion4/1 -> NVSE_RRslipFlag_rat/1  "NVSE_RRslipFlag_rat"
  Data Type Conversion5/1 -> NVSE_LRslipFlag_rat/1  "NVSE_LRslipFlag_rat"
  Data Type Conversion6/1 -> NVSE_RFslipFlag_rat/1  "NVSE_RFslipFlag_rat"
  Data Type Conversion7/1 -> NVSE_LFslipFlag_rat/1  "NVSE_LFslipFlag_rat"

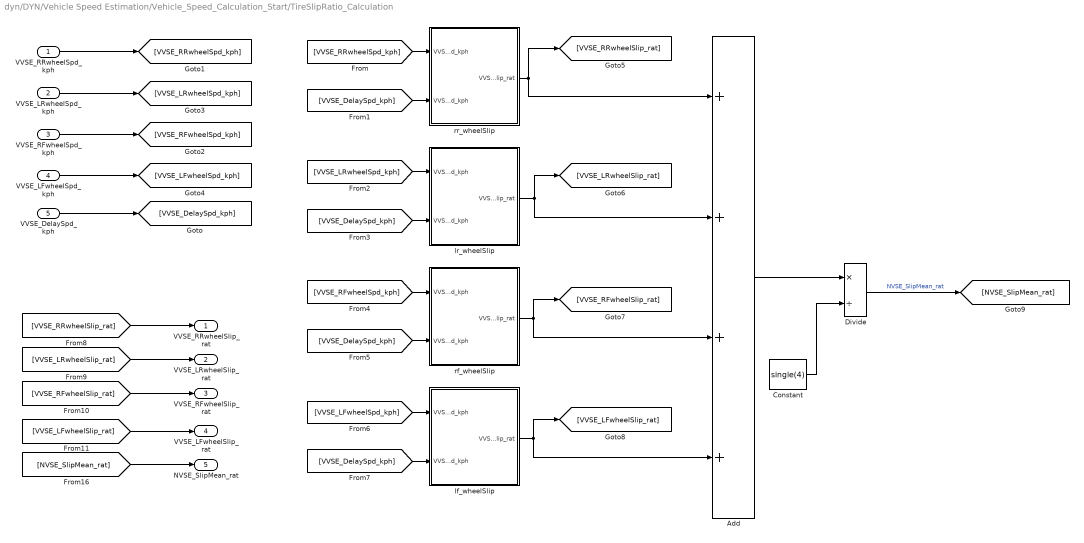
== system dyn/DYN/Vehicle Speed Estimation/Vehicle_Speed_Calculation_Start/TireSlipRatio_Calculation ==
  VVSE_RRwheelSpd_kph : Inport
  VVSE_LRwheelSpd_kph : Inport  Port=2
  VVSE_RFwheelSpd_kph : Inport  Port=3
  VVSE_LFwheelSpd_kph : Inport  Port=4
  VVSE_DelaySpd_kph : Inport  Port=5
  Add : Sum  Inputs=++++
  Constant : Constant  Value=single(4)
  Divide : Product  Inputs=*/
  "lf_wheelSlip " : Subsystem
  lr_wheelSlip : Subsystem
  rf_wheelSlip : Subsystem
  rr_wheelSlip : Subsystem  RequirementInfo={} %GIDa_c8b2f6a2_3d64_4d29_9794_b0dc0d6a5f58
  VVSE_RRwheelSlip_rat : Outport
  VVSE_LRwheelSlip_rat : Outport  Port=2
  VVSE_RFwheelSlip_rat : Outport  Port=3
  VVSE_LFwheelSlip_rat : Outport  Port=4
  NVSE_SlipMean_rat : Outport  Port=5
  wires:
  [VVSE_RRwheelSpd_kph] -> rr_wheelSlip/1(VVSE_RRwheelSpd_kph)
  [VVSE_LFwheelSpd_kph] -> "lf_wheelSlip "/1(VVSE_LFwheelSpd_kph)
  [VVSE_DelaySpd_kph] -> "lf_wheelSlip "/2(VVSE_DelaySpd_kph)
  [VVSE_DelaySpd_kph] -> lr_wheelSlip/2(VVSE_DelaySpd_kph)
  VVSE_LRwheelSpd_kph/1 -> [VVSE_LRwheelSpd_kph]
  VVSE_LFwheelSpd_kph/1 -> [VVSE_LFwheelSpd_kph]
  [VVSE_LRwheelSpd_kph] -> lr_wheelSlip/1(VVSE_LRwheelSpd_kph)
  [VVSE_DelaySpd_kph] -> rf_wheelSlip/2(VVSE_DelaySpd_kph)
  [VVSE_RFwheelSpd_kph] -> rf_wheelSlip/1(VVSE_RFwheelSpd_kph)
  lr_wheelSlip/1(VVSE_LRwheelSlip_rat) -> [VVSE_LRwheelSlip_rat], Add/2
  VVSE_RFwheelSpd_kph/1 -> [VVSE_RFwheelSpd_kph]
  [VVSE_RFwheelSlip_rat] -> VVSE_RFwheelSlip_rat/1
  [VVSE_RRwheelSlip_rat] -> VVSE_RRwheelSlip_rat/1
  rr_wheelSlip/1(VVSE_RRwheelSlip_rat) -> Add/1, [VVSE_RRwheelSlip_rat]
  rf_wheelSlip/1(VVSE_RFwheelSlip_rat) -> Add/3, [VVSE_RFwheelSlip_rat]
  VVSE_RRwheelSpd_kph/1 -> [VVSE_RRwheelSpd_kph]
  [VVSE_LFwheelSlip_rat] -> VVSE_LFwheelSlip_rat/1
  [VVSE_LRwheelSlip_rat] -> VVSE_LRwheelSlip_rat/1
  [VVSE_DelaySpd_kph] -> rr_wheelSlip/2(VVSE_DelaySpd_kph)
  [NVSE_SlipMean_rat] -> NVSE_SlipMean_rat/1
  "lf_wheelSlip "/1(VVSE_LFwheelSlip_rat) -> Add/4, [VVSE_LFwheelSlip_rat]
  Add/1 -> Divide/1
  Divide/1 -> [NVSE_SlipMean_rat]  "NVSE_SlipMean_rat"
  VVSE_DelaySpd_kph/1 -> [VVSE_DelaySpd_kph]
  Constant/1 -> Divide/2

== system dyn/DYN/Vehicle Speed Estimation/Vehicle_Speed_Calculation_Start/WheelSpeed_Mean_Calculation ==
  VVSE_RRwheelSpd_kph : Inport
  NVSE_RRslipFlag_rat : Inport  Port=2
  VVSE_LRwheelSpd_kph : Inport  Port=3
  NVSE_LRslipFlag_rat : Inport  Port=4
  VVSE_RFwheelSpd_kph : Inport  Port=5
  NVSE_RFslipFlag_rat : Inport  Port=6
  VVSE_LFwheelSpd_kph : Inport  Port=7
  NVSE_LFslipFlag_rat : Inport  Port=8
  Add5 : Sum  Inputs=++++
  Add6 : Sum  Inputs=++++
  Bias : Bias  Bias=1e-6
  Divide : Product  Inputs=*/
  Product{,1..3} (4 alike) : Product
  VVSE_VehSpdStart_kph : Outport
  wires:
  NVSE_RRslipFlag_rat/1 -> Add6/1, Product/2
  VVSE_LRwheelSpd_kph/1 -> Product1/1
  NVSE_LRslipFlag_rat/1 -> Add6/2, Product1/2
  Add5/1 -> Divide/1
  VVSE_RFwheelSpd_kph/1 -> Product2/1
  NVSE_RFslipFlag_rat/1 -> Add6/3, Product2/2
  NVSE_LFslipFlag_rat/1 -> Product3/2, Add6/4
  Product3/1 -> Add5/4
  Product2/1 -> Add5/3
  Product1/1 -> Add5/2
  Product/1 -> Add5/1
  Add6/1 -> Bias/1
  Bias/1 -> Divide/2
  VVSE_RRwheelSpd_kph/1 -> Product/1
  VVSE_LFwheelSpd_kph/1 -> Product3/1
  Divide/1 -> VVSE_VehSpdStart_kph/1  "VVSE_VehSpdStart_kph"

== system dyn/DYN/Vehicle Speed Estimation/Vehicle_Speed_Calculation_Turn /Speed_Calculation1 ==
  VVSE_RRwheelPercent_pct : Inport
  VVSE_RRwheelSpd_kph : Inport  Port=2
  VVSE_LRwheelPercent_pct : Inport  Port=3
  VVSE_LRwheelSpd_kph : Inport  Port=4
  VVSE_RFwheelPercent_pct : Inport  Port=5
  VVSE_RFwheelSpd_kph : Inport  Port=6
  VVSE_LFwheelPercent_pct : Inport  Port=7
  VVSE_LFwheelSpd_kph : Inport  Port=8
  VVSE_AccelPercent_pct : Inport  Port=9
  VVSE_LongAccel_G : Inport  Port=10
  VVSE_DelaySpd_kph : Inport  Port=11
  Add : Sum
  Add1 : Sum  Inputs=+++++
  Gain : Gain  Gain=9.81
  Gain1 : Gain  Gain=0.01
  Gain2 : Gain  Gain=3.6
  Product{,1..4} (5 alike) : Product
  VVSE_VehSpdTurn_kph : Outport
  wires:
  Gain/1 -> Gain1/1
  Product4/1 -> Add1/5
  Product/1 -> Add1/1
  Add/1 -> Product4/2
  Product1/1 -> Add1/2
  Product2/1 -> Add1/3
  Gain2/1 -> Add/1
  Product3/1 -> Add1/4
  Gain1/1 -> Gain2/1
  VVSE_RRwheelPercent_pct/1 -> Product/1
  VVSE_RFwheelPercent_pct/1 -> Product2/1
  VVSE_LongAccel_G/1 -> Gain/1
  VVSE_DelaySpd_kph/1 -> Add/2
  VVSE_LRwheelPercent_pct/1 -> Product1/1
  VVSE_LRwheelSpd_kph/1 -> Product1/2
  VVSE_AccelPercent_pct/1 -> Product4/1
  VVSE_LFwheelSpd_kph/1 -> Product3/2
  VVSE_RRwheelSpd_kph/1 -> Product/2
  VVSE_RFwheelSpd_kph/1 -> Product2/2
  VVSE_LFwheelPercent_pct/1 -> Product3/1
  Add1/1 -> VVSE_VehSpdTurn_kph/1  "VVSE_VehSpdTurn_kph"

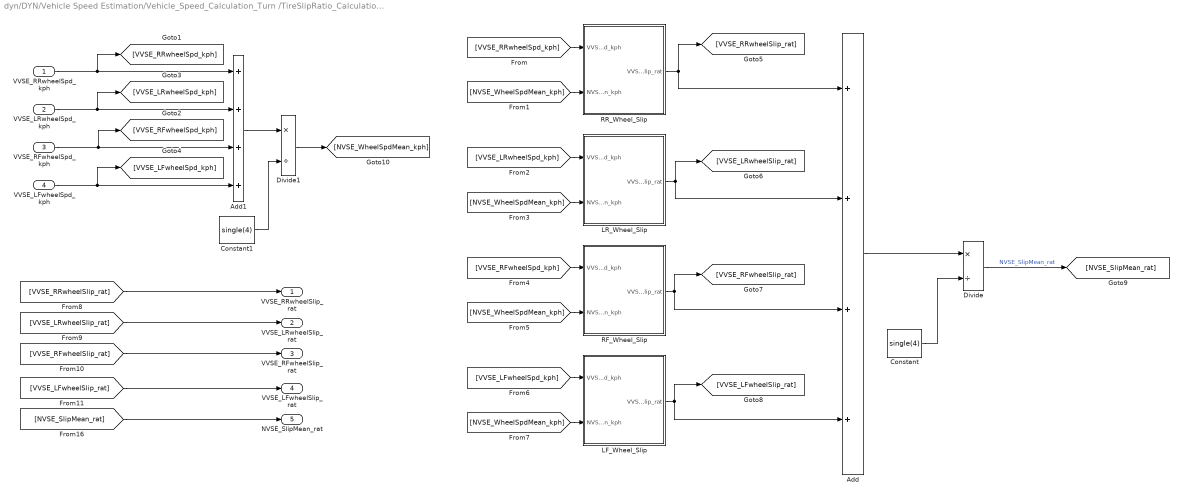
== system dyn/DYN/Vehicle Speed Estimation/Vehicle_Speed_Calculation_Turn /TireSlipRatio_Calculation1 ==
  VVSE_RRwheelSpd_kph : Inport
  VVSE_LRwheelSpd_kph : Inport  Port=2
  VVSE_RFwheelSpd_kph : Inport  Port=3
  VVSE_LFwheelSpd_kph : Inport  Port=4
  Add : Sum  Inputs=++++
  Add1 : Sum  Inputs=++++
  Constant : Constant  Value=single(4)
  Constant1 : Constant  Value=single(4)
  Divide : Product  Inputs=*/
  Divide1 : Product  Inputs=*/
  "LF_Wheel_Slip " : Subsystem
  LR_Wheel_Slip : Subsystem
  RF_Wheel_Slip : Subsystem
  RR_Wheel_Slip : Subsystem  RequirementInfo={} %GIDa_c8b2f6a2_3d64_4d29_9794_b0dc0d6a5f58
  VVSE_RRwheelSlip_rat : Outport
  VVSE_LRwheelSlip_rat : Outport  Port=2
  VVSE_RFwheelSlip_rat : Outport  Port=3
  VVSE_LFwheelSlip_rat : Outport  Port=4
  NVSE_SlipMean_rat : Outport  Port=5
  wires:
  [VVSE_RRwheelSpd_kph] -> RR_Wheel_Slip/1(VVSE_RRwheelSpd_kph)
  [VVSE_LFwheelSpd_kph] -> "LF_Wheel_Slip "/1(VVSE_LFwheelSpd_kph)
  [NVSE_WheelSpdMean_kph] -> "LF_Wheel_Slip "/2(NVSE_WheelSpdMean_kph)
  [NVSE_WheelSpdMean_kph] -> LR_Wheel_Slip/2(NVSE_WheelSpdMean_kph)
  VVSE_LRwheelSpd_kph/1 -> [VVSE_LRwheelSpd_kph], Add1/2
  VVSE_LFwheelSpd_kph/1 -> [VVSE_LFwheelSpd_kph], Add1/4
  [VVSE_LRwheelSpd_kph] -> LR_Wheel_Slip/1(VVSE_LRwheelSpd_kph)
  [NVSE_WheelSpdMean_kph] -> RF_Wheel_Slip/2(NVSE_WheelSpdMean_kph)
  [VVSE_RFwheelSpd_kph] -> RF_Wheel_Slip/1(VVSE_RFwheelSpd_kph)
  LR_Wheel_Slip/1(VVSE_LRwheelSlip_rat) -> [VVSE_LRwheelSlip_rat], Add/2
  VVSE_RFwheelSpd_kph/1 -> [VVSE_RFwheelSpd_kph], Add1/3
  [VVSE_RFwheelSlip_rat] -> VVSE_RFwheelSlip_rat/1
  [VVSE_RRwheelSlip_rat] -> VVSE_RRwheelSlip_rat/1
  RR_Wheel_Slip/1(VVSE_RRwheelSlip_rat) -> Add/1, [VVSE_RRwheelSlip_rat]
  RF_Wheel_Slip/1(VVSE_RFwheelSlip_rat) -> Add/3, [VVSE_RFwheelSlip_rat]
  VVSE_RRwheelSpd_kph/1 -> [VVSE_RRwheelSpd_kph], Add1/1
  [VVSE_LFwheelSlip_rat] -> VVSE_LFwheelSlip_rat/1
  [VVSE_LRwheelSlip_rat] -> VVSE_LRwheelSlip_rat/1
  [NVSE_WheelSpdMean_kph] -> RR_Wheel_Slip/2(NVSE_WheelSpdMean_kph)
  [NVSE_SlipMean_rat] -> NVSE_SlipMean_rat/1
  "LF_Wheel_Slip "/1(VVSE_LFwheelSlip_rat) -> Add/4, [VVSE_LFwheelSlip_rat]
  Add/1 -> Divide/1
  Divide/1 -> [NVSE_SlipMean_rat]  "NVSE_SlipMean_rat"
  Constant/1 -> Divide/2
  Divide1/1 -> [NVSE_WheelSpdMean_kph]
  Constant1/1 -> Divide1/2
  Add1/1 -> Divide1/1

== system dyn/DYN/Vehicle Speed Estimation/Vehicle_Speed_Calculation_Turn /Weight_Calculation ==
  VVSE_RRwheelSlip_rat : Inport
  VVSE_LRwheelSlip_rat : Inport  Port=2
  VVSE_RFwheelSlip_rat : Inport  Port=3
  VVSE_LFwheelSlip_rat : Inport  Port=4
  NVSE_SlipMean_rat : Inport  Port=5
  VVSE_LongAccel_G : Inport  Port=6
  Percentage : Subsystem  RequirementInfo={} %GIDa_b7f10889_7b75_40d3_8cb6_4d2c6f0c621d
  Weight : Subsystem  RequirementInfo={} %GIDa_ee7ecb5e_3ba9_4a62_b515_b78ff1211ee4
  VVSE_RRwheelPercent_pct : Outport
  VVSE_LRwheelPercent_pct : Outport  Port=2
  VVSE_RFwheelPercent_pct : Outport  Port=3
  VVSE_LFwheelPercent_pct : Outport  Port=4
  VVSE_AccelPercent_pct : Outport  Port=5
  wires:
  NVSE_SlipMean_rat/1 -> Weight/5(NVSE_SlipMean_rat)
  Weight/5(NVSE_AccelWeight_rat) -> Percentage/5(NVSE_AccelWeight_rat)
  Weight/4(NVSE_LFwheelWeight_rat) -> Percentage/4(NVSE_LFwheelWeight_rat)
  Weight/3(NVSE_RFwheelWeight_rat) -> Percentage/3(NVSE_RFwheelWeight_rat)
  Weight/2(NVSE_LRwheelWeight_rat) -> Percentage/2(NVSE_LRwheelWeight_rat)
  Weight/1(NVSE_RRwheelWeight_rat) -> Percentage/1(NVSE_RRwheelWeight_rat)
  VVSE_LongAccel_G/1 -> Weight/6(VVSE_LongAccel_G)
  VVSE_LFwheelSlip_rat/1 -> Weight/4(VVSE_LFwheelSlip_rat)
  VVSE_RFwheelSlip_rat/1 -> Weight/3(VVSE_RFwheelSlip_rat)
  VVSE_LRwheelSlip_rat/1 -> Weight/2(VVSE_LRwheelSlip_rat)
  VVSE_RRwheelSlip_rat/1 -> Weight/1(VVSE_RRwheelSlip_rat)
  Percentage/5(VVSE_AccelPercent_pct) -> VVSE_AccelPercent_pct/1
  Percentage/4(VVSE_LFwheelPercent_pct) -> VVSE_LFwheelPercent_pct/1
  Percentage/3(VVSE_RFwheelPercent_pct) -> VVSE_RFwheelPercent_pct/1
  Percentage/2(VVSE_LRwheelPercent_pct) -> VVSE_LRwheelPercent_pct/1
  Percentage/1(VVSE_RRwheelPercent_pct) -> VVSE_RRwheelPercent_pct/1

== system dyn/DYN/Vehicle Speed Estimation/Vehicle_Speed_Calculation_Normal /TireSlipRatio_Calculation/LF_Wheel_Slip  ==
  VVSE_LFwheelSpd_kph : Inport
  VVSE_DelaySpd_kph : Inport  Port=2
  Add : Sum  Inputs=+-
  Add1 : Sum  Inputs=+-
  Bias : Bias  Bias=1e-6
  Bias1 : Bias  Bias=1e-6
  Divide : Product  Inputs=*/
  Divide1 : Product  Inputs=*/
  Gain : Gain  Gain=-1
  Switch : Switch  Criteria=u2 > Threshold
  VVSE_LFwheelSlip_rat : Outport
  wires:
  Divide/1 -> Switch/1
  Divide1/1 -> Switch/3
  Switch/1 -> VVSE_LFwheelSlip_rat/1  "VVSE_LFwheelSlip_rat"
  [VVSE_DelaySpd_kph] -> Bias1/1
  [VVSE_LFwheelSpd_kph] -> Add/1
  [VVSE_LFwheelSpd_kph] -> Bias/1
  Add/1 -> Divide/1
  Bias/1 -> Divide/2
  VVSE_DelaySpd_kph/1 -> [VVSE_DelaySpd_kph]
  VVSE_LFwheelSpd_kph/1 -> [VVSE_LFwheelSpd_kph]
  Gain/1 -> Divide1/1
  [VVSE_DelaySpd_kph] -> Add/2
  Add1/1 -> Switch/2, Gain/1
  [VVSE_DelaySpd_kph] -> Add1/2
  [VVSE_LFwheelSpd_kph] -> Add1/1
  Bias1/1 -> Divide1/2

== system dyn/DYN/Vehicle Speed Estimation/Vehicle_Speed_Calculation_Normal /TireSlipRatio_Calculation/LR_Wheel_Slip ==
  VVSE_LRwheelSpd_kph : Inport
  VVSE_DelaySpd_kph : Inport  Port=2
  Add : Sum  Inputs=+-
  Add1 : Sum  Inputs=+-
  Bias : Bias  Bias=1e-6
  Bias1 : Bias  Bias=1e-6
  Divide : Product  Inputs=*/
  Divide1 : Product  Inputs=*/
  Gain : Gain  Gain=-1
  Switch : Switch  Criteria=u2 > Threshold
  VVSE_LRwheelSlip_rat : Outport
  wires:
  Divide1/1 -> Switch/3
  Divide/1 -> Switch/1
  Switch/1 -> VVSE_LRwheelSlip_rat/1  "VVSE_LRwheelSlip_rat"
  [VVSE_LRwheelSpd_kph] -> Add/1
  [VVSE_LRwheelSpd_kph] -> Bias/1
  Add/1 -> Divide/1
  Bias/1 -> Divide/2
  VVSE_DelaySpd_kph/1 -> [VVSE_DelaySpd_kph]
  VVSE_LRwheelSpd_kph/1 -> [VVSE_LRwheelSpd_kph]
  Gain/1 -> Divide1/1
  [VVSE_DelaySpd_kph] -> Bias1/1
  [VVSE_DelaySpd_kph] -> Add/2
  Add1/1 -> Gain/1, Switch/2
  [VVSE_DelaySpd_kph] -> Add1/2
  [VVSE_LRwheelSpd_kph] -> Add1/1
  Bias1/1 -> Divide1/2

== system dyn/DYN/Vehicle Speed Estimation/Vehicle_Speed_Calculation_Normal /TireSlipRatio_Calculation/RF_Wheel_Slip ==
  VVSE_RFwheelSpd_kph : Inport
  VVSE_DelaySpd_kph : Inport  Port=2
  Add : Sum  Inputs=+-
  Add1 : Sum  Inputs=+-
  Bias : Bias  Bias=1e-6
  Bias2 : Bias  Bias=1e-6
  Divide : Product  Inputs=*/
  Divide1 : Product  Inputs=*/
  Gain : Gain  Gain=-1
  Switch : Switch  Criteria=u2 > Threshold
  VVSE_RFwheelSlip_rat : Outport
  wires:
  Divide/1 -> Switch/1
  Divide1/1 -> Switch/3
  Switch/1 -> VVSE_RFwheelSlip_rat/1  "VVSE_RFwheelSlip_rat"
  Bias2/1 -> Divide1/2
  [VVSE_RFwheelSpd_kph] -> Add1/1
  [VVSE_DelaySpd_kph] -> Add1/2
  Add1/1 -> Switch/2, Gain/1
  [VVSE_DelaySpd_kph] -> Add/2
  [VVSE_DelaySpd_kph] -> Bias2/1
  Gain/1 -> Divide1/1
  VVSE_RFwheelSpd_kph/1 -> [VVSE_RFwheelSpd_kph]
  VVSE_DelaySpd_kph/1 -> [VVSE_DelaySpd_kph]
  Bias/1 -> Divide/2
  Add/1 -> Divide/1
  [VVSE_RFwheelSpd_kph] -> Bias/1
  [VVSE_RFwheelSpd_kph] -> Add/1

== system dyn/DYN/Vehicle Speed Estimation/Vehicle_Speed_Calculation_Normal /TireSlipRatio_Calculation/RR_Wheel_Slip ==
  VVSE_RRwheelSpd_kph : Inport
  VVSE_DelaySpd_kph : Inport  Port=2
  Add : Sum  Inputs=+-
  Add1 : Sum  Inputs=+-
  Bias : Bias  Bias=1e-6
  Bias1 : Bias  Bias=1e-6
  Divide : Product  Inputs=*/
  Divide1 : Product  Inputs=*/
  Gain : Gain  Gain=-1
  Switch : Switch  Criteria=u2 > Threshold
  VVSE_RRwheelSlip_rat : Outport
  wires:
  Divide1/1 -> Switch/3
  Divide/1 -> Switch/1
  Switch/1 -> VVSE_RRwheelSlip_rat/1  "VVSE_RRwheelSlip_rat"
  Bias1/1 -> Divide1/2
  [VVSE_RRwheelSpd_kph] -> Add1/1
  [VVSE_DelaySpd_kph] -> Add1/2
  Add1/1 -> Gain/1, Switch/2
  [VVSE_DelaySpd_kph] -> Add/2
  [VVSE_DelaySpd_kph] -> Bias1/1
  Gain/1 -> Divide1/1
  VVSE_RRwheelSpd_kph/1 -> [VVSE_RRwheelSpd_kph]
  VVSE_DelaySpd_kph/1 -> [VVSE_DelaySpd_kph]
  Bias/1 -> Divide/2
  Add/1 -> Divide/1
  [VVSE_RRwheelSpd_kph] -> Bias/1
  [VVSE_RRwheelSpd_kph] -> Add/1

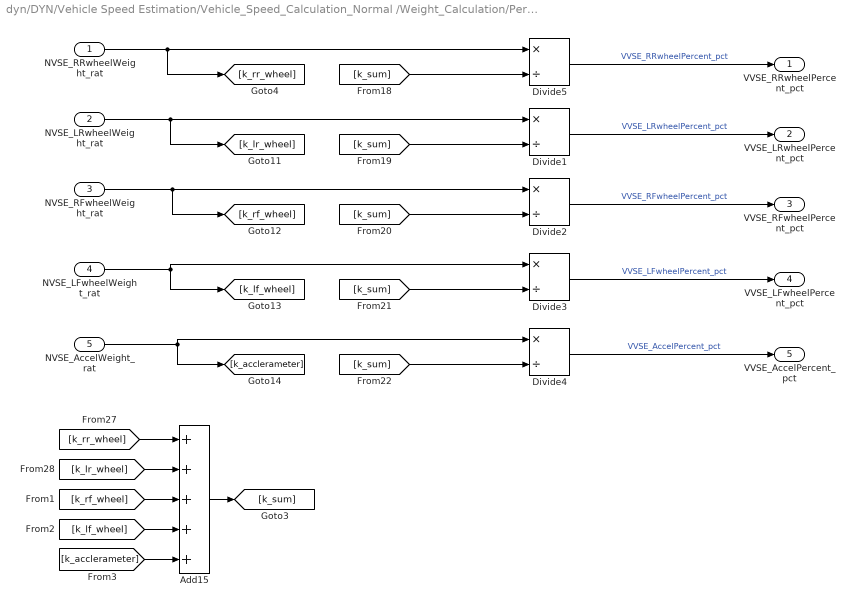
== system dyn/DYN/Vehicle Speed Estimation/Vehicle_Speed_Calculation_Normal /Weight_Calculation/Percentage ==
  NVSE_RRwheelWeight_rat : Inport
  NVSE_LRwheelWeight_rat : Inport  Port=2
  NVSE_RFwheelWeight_rat : Inport  Port=3
  NVSE_LFwheelWeight_rat : Inport  Port=4
  NVSE_AccelWeight_rat : Inport  Port=5
  Add15 : Sum  Inputs=+++++
  Divide{1..5} (5 alike) : Product  Inputs=*/
  VVSE_RRwheelPercent_pct : Outport
  VVSE_LRwheelPercent_pct : Outport  Port=2
  VVSE_RFwheelPercent_pct : Outport  Port=3
  VVSE_LFwheelPercent_pct : Outport  Port=4
  VVSE_AccelPercent_pct : Outport  Port=5
  wires:
  NVSE_LFwheelWeight_rat/1 -> Divide3/1, [k_lf_wheel]
  NVSE_AccelWeight_rat/1 -> Divide4/1, [k_acclerameter]
  Divide3/1 -> VVSE_LFwheelPercent_pct/1  "VVSE_LFwheelPercent_pct"
  Divide2/1 -> VVSE_RFwheelPercent_pct/1  "VVSE_RFwheelPercent_pct"
  NVSE_RRwheelWeight_rat/1 -> Divide5/1, [k_rr_wheel]
  NVSE_LRwheelWeight_rat/1 -> Divide1/1, [k_lr_wheel]
  [k_sum] -> Divide5/2
  Divide4/1 -> VVSE_AccelPercent_pct/1  "VVSE_AccelPercent_pct"
  Divide1/1 -> VVSE_LRwheelPercent_pct/1  "VVSE_LRwheelPercent_pct"
  Divide5/1 -> VVSE_RRwheelPercent_pct/1  "VVSE_RRwheelPercent_pct"
  NVSE_RFwheelWeight_rat/1 -> Divide2/1, [k_rf_wheel]
  [k_rr_wheel] -> Add15/1
  [k_lr_wheel] -> Add15/2
  [k_rf_wheel] -> Add15/3
  [k_lf_wheel] -> Add15/4
  [k_acclerameter] -> Add15/5
  Add15/1 -> [k_sum]
  [k_sum] -> Divide4/2
  [k_sum] -> Divide2/2
  [k_sum] -> Divide3/2
  [k_sum] -> Divide1/2

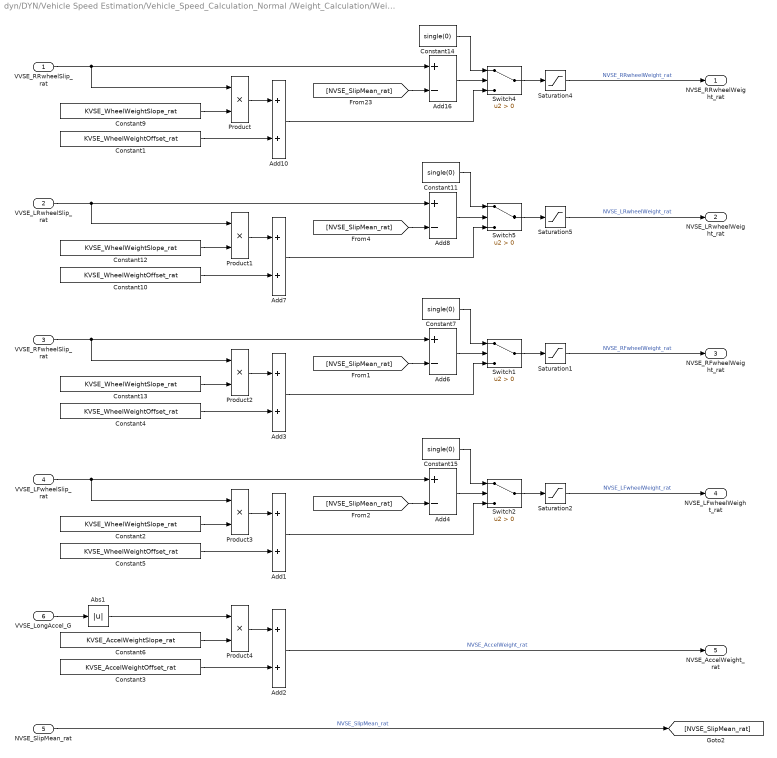
== system dyn/DYN/Vehicle Speed Estimation/Vehicle_Speed_Calculation_Normal /Weight_Calculation/Weight ==
  VVSE_RRwheelSlip_rat : Inport
  VVSE_LRwheelSlip_rat : Inport  Port=2
  VVSE_RFwheelSlip_rat : Inport  Port=3
  VVSE_LFwheelSlip_rat : Inport  Port=4
  NVSE_SlipMean_rat : Inport  Port=5
  VVSE_LongAccel_G : Inport  Port=6
  Abs1 : Abs
  Add{1..3,7,10} (5 alike) : Sum
  Add{4,6,8,16} (4 alike) : Sum  Inputs=+-
  Constant{1,4..5,10} (4 alike) : Constant  Value=KVSE_WheelWeightOffset_rat
  Constant{7,11,14..15} (4 alike) : Constant  Value=single(0)
  Constant{2,9,12..13} (4 alike) : Constant  Value=KVSE_WheelWeightSlope_rat
  Constant3 : Constant  Value=KVSE_AccelWeightOffset_rat
  Constant6 : Constant  Value=KVSE_AccelWeightSlope_rat
  Product{,1..4} (5 alike) : Product
  Saturation{1..2,4..5} (4 alike) : Saturate  UpperLimit=Inf  LowerLimit=0
  Switch{1..2,4..5} (4 alike) : Switch  Criteria=u2 > Threshold
  NVSE_RRwheelWeight_rat : Outport
  NVSE_LRwheelWeight_rat : Outport  Port=2
  NVSE_RFwheelWeight_rat : Outport  Port=3
  NVSE_LFwheelWeight_rat : Outport  Port=4
  NVSE_AccelWeight_rat : Outport  Port=5
  wires:
  VVSE_LongAccel_G/1 -> Abs1/1
  [NVSE_SlipMean_rat] -> Add16/2
  NVSE_SlipMean_rat/1 -> [NVSE_SlipMean_rat]  "NVSE_SlipMean_rat"
  Abs1/1 -> Product4/1
  Add16/1 -> Switch4/2
  Add10/1 -> Switch4/3
  Constant14/1 -> Switch4/1
  Add2/1 -> NVSE_AccelWeight_rat/1  "NVSE_AccelWeight_rat"
  Product/1 -> Add10/1
  Constant1/1 -> Add10/2
  VVSE_RRwheelSlip_rat/1 -> Product/1, Add16/1
  Saturation4/1 -> NVSE_RRwheelWeight_rat/1  "NVSE_RRwheelWeight_rat"
  Switch4/1 -> Saturation4/1
  Constant3/1 -> Add2/2
  Constant9/1 -> Product/2
  [NVSE_SlipMean_rat] -> Add8/2
  Add8/1 -> Switch5/2
  Add7/1 -> Switch5/3
  Constant11/1 -> Switch5/1
  Product1/1 -> Add7/1
  Constant10/1 -> Add7/2
  VVSE_LRwheelSlip_rat/1 -> Product1/1, Add8/1
  Saturation5/1 -> NVSE_LRwheelWeight_rat/1  "NVSE_LRwheelWeight_rat"
  Switch5/1 -> Saturation5/1
  Constant12/1 -> Product1/2
  [NVSE_SlipMean_rat] -> Add6/2
  Add6/1 -> Switch1/2
  Add3/1 -> Switch1/3
  Constant7/1 -> Switch1/1
  Product2/1 -> Add3/1
  Constant4/1 -> Add3/2
  VVSE_RFwheelSlip_rat/1 -> Product2/1, Add6/1
  Saturation1/1 -> NVSE_RFwheelWeight_rat/1  "NVSE_RFwheelWeight_rat"
  Switch1/1 -> Saturation1/1
  Constant13/1 -> Product2/2
  [NVSE_SlipMean_rat] -> Add4/2
  Add4/1 -> Switch2/2
  Add1/1 -> Switch2/3
  Constant15/1 -> Switch2/1
  Product3/1 -> Add1/1
  Constant5/1 -> Add1/2
  VVSE_LFwheelSlip_rat/1 -> Product3/1, Add4/1
  Saturation2/1 -> NVSE_LFwheelWeight_rat/1  "NVSE_LFwheelWeight_rat"
  Switch2/1 -> Saturation2/1
  Constant2/1 -> Product3/2
  Product4/1 -> Add2/1
  Constant6/1 -> Product4/2

== system dyn/DYN/Vehicle Speed Estimation/Vehicle_Speed_Calculation_Start/TireSlipRatio_Calculation/lf_wheelSlip  ==
  VVSE_LFwheelSpd_kph : Inport
  VVSE_DelaySpd_kph : Inport  Port=2
  Add : Sum  Inputs=+-
  Add1 : Sum  Inputs=+-
  Bias : Bias  Bias=1e-6
  Bias1 : Bias  Bias=1e-6
  Divide : Product  Inputs=*/
  Divide1 : Product  Inputs=*/
  Gain : Gain  Gain=-1
  Switch : Switch  Criteria=u2 > Threshold
  VVSE_LFwheelSlip_rat : Outport
  wires:
  Bias1/1 -> Divide1/2
  [VVSE_LFwheelSpd_kph] -> Add1/1
  [VVSE_DelaySpd_kph] -> Add1/2
  Add1/1 -> Gain/1, Switch/2
  [VVSE_DelaySpd_kph] -> Add/2
  Gain/1 -> Divide1/1
  VVSE_LFwheelSpd_kph/1 -> [VVSE_LFwheelSpd_kph]
  VVSE_DelaySpd_kph/1 -> [VVSE_DelaySpd_kph]
  Bias/1 -> Divide/2
  Add/1 -> Divide/1
  [VVSE_LFwheelSpd_kph] -> Bias/1
  [VVSE_LFwheelSpd_kph] -> Add/1
  [VVSE_DelaySpd_kph] -> Bias1/1
  Switch/1 -> VVSE_LFwheelSlip_rat/1  "VVSE_LFwheelSlip_rat"
  Divide1/1 -> Switch/3
  Divide/1 -> Switch/1

== system dyn/DYN/Vehicle Speed Estimation/Vehicle_Speed_Calculation_Start/TireSlipRatio_Calculation/lr_wheelSlip ==
  VVSE_LRwheelSpd_kph : Inport
  VVSE_DelaySpd_kph : Inport  Port=2
  Add : Sum  Inputs=+-
  Add1 : Sum  Inputs=+-
  Bias : Bias  Bias=1e-6
  Bias1 : Bias  Bias=1e-6
  Divide : Product  Inputs=*/
  Divide1 : Product  Inputs=*/
  Gain : Gain  Gain=-1
  Switch : Switch  Criteria=u2 > Threshold
  VVSE_LRwheelSlip_rat : Outport
  wires:
  Bias1/1 -> Divide1/2
  [VVSE_LRwheelSpd_kph] -> Add1/1
  [VVSE_DelaySpd_kph] -> Add1/2
  Add1/1 -> Switch/2, Gain/1
  [VVSE_DelaySpd_kph] -> Add/2
  [VVSE_DelaySpd_kph] -> Bias1/1
  Gain/1 -> Divide1/1
  VVSE_LRwheelSpd_kph/1 -> [VVSE_LRwheelSpd_kph]
  VVSE_DelaySpd_kph/1 -> [VVSE_DelaySpd_kph]
  Bias/1 -> Divide/2
  Add/1 -> Divide/1
  [VVSE_LRwheelSpd_kph] -> Bias/1
  [VVSE_LRwheelSpd_kph] -> Add/1
  Switch/1 -> VVSE_LRwheelSlip_rat/1  "VVSE_LRwheelSlip_rat"
  Divide/1 -> Switch/1
  Divide1/1 -> Switch/3

== system dyn/DYN/Vehicle Speed Estimation/Vehicle_Speed_Calculation_Start/TireSlipRatio_Calculation/rf_wheelSlip ==
  VVSE_RFwheelSpd_kph : Inport
  VVSE_DelaySpd_kph : Inport  Port=2
  Add : Sum  Inputs=+-
  Add1 : Sum  Inputs=+-
  Bias : Bias  Bias=1e-6
  Bias2 : Bias  Bias=1e-6
  Divide : Product  Inputs=*/
  Divide1 : Product  Inputs=*/
  Gain : Gain  Gain=-1
  Switch : Switch  Criteria=u2 > Threshold
  VVSE_RFwheelSlip_rat : Outport
  wires:
  [VVSE_RFwheelSpd_kph] -> Add/1
  [VVSE_RFwheelSpd_kph] -> Bias/1
  Add/1 -> Divide/1
  Bias/1 -> Divide/2
  VVSE_DelaySpd_kph/1 -> [VVSE_DelaySpd_kph]
  VVSE_RFwheelSpd_kph/1 -> [VVSE_RFwheelSpd_kph]
  Gain/1 -> Divide1/1
  [VVSE_DelaySpd_kph] -> Bias2/1
  [VVSE_DelaySpd_kph] -> Add/2
  Add1/1 -> Gain/1, Switch/2
  [VVSE_DelaySpd_kph] -> Add1/2
  [VVSE_RFwheelSpd_kph] -> Add1/1
  Bias2/1 -> Divide1/2
  Switch/1 -> VVSE_RFwheelSlip_rat/1  "VVSE_RFwheelSlip_rat"
  Divide1/1 -> Switch/3
  Divide/1 -> Switch/1

== system dyn/DYN/Vehicle Speed Estimation/Vehicle_Speed_Calculation_Start/TireSlipRatio_Calculation/rr_wheelSlip ==
  VVSE_RRwheelSpd_kph : Inport
  VVSE_DelaySpd_kph : Inport  Port=2
  Add : Sum  Inputs=+-
  Add1 : Sum  Inputs=+-
  Bias : Bias  Bias=1e-6
  Bias1 : Bias  Bias=1e-6
  Divide : Product  Inputs=*/
  Divide1 : Product  Inputs=*/
  Gain : Gain  Gain=-1
  Switch : Switch  Criteria=u2 > Threshold
  VVSE_RRwheelSlip_rat : Outport
  wires:
  [VVSE_RRwheelSpd_kph] -> Add/1
  [VVSE_RRwheelSpd_kph] -> Bias/1
  Add/1 -> Divide/1
  Bias/1 -> Divide/2
  VVSE_DelaySpd_kph/1 -> [VVSE_DelaySpd_kph]
  VVSE_RRwheelSpd_kph/1 -> [VVSE_RRwheelSpd_kph]
  Gain/1 -> Divide1/1
  [VVSE_DelaySpd_kph] -> Bias1/1
  [VVSE_DelaySpd_kph] -> Add/2
  Add1/1 -> Switch/2, Gain/1
  [VVSE_DelaySpd_kph] -> Add1/2
  [VVSE_RRwheelSpd_kph] -> Add1/1
  Bias1/1 -> Divide1/2
  Switch/1 -> VVSE_RRwheelSlip_rat/1  "VVSE_RRwheelSlip_rat"
  Divide/1 -> Switch/1
  Divide1/1 -> Switch/3

== system dyn/DYN/Vehicle Speed Estimation/Vehicle_Speed_Calculation_Turn /TireSlipRatio_Calculation1/LF_Wheel_Slip  ==
  VVSE_LFwheelSpd_kph : Inport
  NVSE_WheelSpdMean_kph : Inport  Port=2
  Add : Sum  Inputs=+-
  Add1 : Sum  Inputs=+-
  Bias : Bias  Bias=1e-6
  Bias1 : Bias  Bias=1e-6
  Divide : Product  Inputs=*/
  Divide1 : Product  Inputs=*/
  Gain : Gain  Gain=-1
  Switch : Switch  Criteria=u2 > Threshold
  VVSE_LFwheelSlip_rat : Outport
  wires:
  Bias1/1 -> Divide1/2
  [VVSE_LFwheelSpd_kph] -> Add1/1
  [NVSE_WheelSpdMean_kph] -> Add1/2
  Add1/1 -> Gain/1, Switch/2
  [NVSE_WheelSpdMean_kph] -> Add/2
  Gain/1 -> Divide1/1
  VVSE_LFwheelSpd_kph/1 -> [VVSE_LFwheelSpd_kph]
  NVSE_WheelSpdMean_kph/1 -> [NVSE_WheelSpdMean_kph]
  Bias/1 -> Divide/2
  Add/1 -> Divide/1
  [VVSE_LFwheelSpd_kph] -> Bias/1
  [VVSE_LFwheelSpd_kph] -> Add/1
  [NVSE_WheelSpdMean_kph] -> Bias1/1
  Switch/1 -> VVSE_LFwheelSlip_rat/1  "VVSE_LFwheelSlip_rat"
  Divide1/1 -> Switch/3
  Divide/1 -> Switch/1

== system dyn/DYN/Vehicle Speed Estimation/Vehicle_Speed_Calculation_Turn /TireSlipRatio_Calculation1/LR_Wheel_Slip ==
  VVSE_LRwheelSpd_kph : Inport
  NVSE_WheelSpdMean_kph : Inport  Port=2
  Add : Sum  Inputs=+-
  Add1 : Sum  Inputs=+-
  Bias : Bias  Bias=1e-6
  Bias1 : Bias  Bias=1e-6
  Divide : Product  Inputs=*/
  Divide1 : Product  Inputs=*/
  Gain : Gain  Gain=-1
  Switch : Switch  Criteria=u2 > Threshold
  VVSE_LRwheelSlip_rat : Outport
  wires:
  Bias1/1 -> Divide1/2
  [VVSE_LRwheelSpd_kph] -> Add1/1
  [NVSE_WheelSpdMean_kph] -> Add1/2
  Add1/1 -> Switch/2, Gain/1
  [NVSE_WheelSpdMean_kph] -> Add/2
  [NVSE_WheelSpdMean_kph] -> Bias1/1
  Gain/1 -> Divide1/1
  VVSE_LRwheelSpd_kph/1 -> [VVSE_LRwheelSpd_kph]
  NVSE_WheelSpdMean_kph/1 -> [NVSE_WheelSpdMean_kph]
  Bias/1 -> Divide/2
  Add/1 -> Divide/1
  [VVSE_LRwheelSpd_kph] -> Bias/1
  [VVSE_LRwheelSpd_kph] -> Add/1
  Switch/1 -> VVSE_LRwheelSlip_rat/1  "VVSE_LRwheelSlip_rat"
  Divide/1 -> Switch/1
  Divide1/1 -> Switch/3

== system dyn/DYN/Vehicle Speed Estimation/Vehicle_Speed_Calculation_Turn /TireSlipRatio_Calculation1/RF_Wheel_Slip ==
  VVSE_RFwheelSpd_kph : Inport
  NVSE_WheelSpdMean_kph : Inport  Port=2
  Add : Sum  Inputs=+-
  Add1 : Sum  Inputs=+-
  Bias : Bias  Bias=1e-6
  Bias2 : Bias  Bias=1e-6
  Divide : Product  Inputs=*/
  Divide1 : Product  Inputs=*/
  Gain : Gain  Gain=-1
  Switch : Switch  Criteria=u2 > Threshold
  VVSE_RFwheelSlip_rat : Outport
  wires:
  [VVSE_RFwheelSpd_kph] -> Add/1
  [VVSE_RFwheelSpd_kph] -> Bias/1
  Add/1 -> Divide/1
  Bias/1 -> Divide/2
  NVSE_WheelSpdMean_kph/1 -> [NVSE_WheelSpdMean_kph]
  VVSE_RFwheelSpd_kph/1 -> [VVSE_RFwheelSpd_kph]
  Gain/1 -> Divide1/1
  [NVSE_WheelSpdMean_kph] -> Bias2/1
  [NVSE_WheelSpdMean_kph] -> Add/2
  Add1/1 -> Gain/1, Switch/2
  [NVSE_WheelSpdMean_kph] -> Add1/2
  [VVSE_RFwheelSpd_kph] -> Add1/1
  Bias2/1 -> Divide1/2
  Switch/1 -> VVSE_RFwheelSlip_rat/1  "VVSE_RFwheelSlip_rat"
  Divide1/1 -> Switch/3
  Divide/1 -> Switch/1

== system dyn/DYN/Vehicle Speed Estimation/Vehicle_Speed_Calculation_Turn /TireSlipRatio_Calculation1/RR_Wheel_Slip ==
  VVSE_RRwheelSpd_kph : Inport
  NVSE_WheelSpdMean_kph : Inport  Port=2
  Add : Sum  Inputs=+-
  Add1 : Sum  Inputs=+-
  Bias : Bias  Bias=1e-6
  Bias1 : Bias  Bias=1e-6
  Divide : Product  Inputs=*/
  Divide1 : Product  Inputs=*/
  Gain : Gain  Gain=-1
  Switch : Switch  Criteria=u2 > Threshold
  VVSE_RRwheelSlip_rat : Outport
  wires:
  [VVSE_RRwheelSpd_kph] -> Add/1
  [VVSE_RRwheelSpd_kph] -> Bias/1
  Add/1 -> Divide/1
  Bias/1 -> Divide/2
  NVSE_WheelSpdMean_kph/1 -> [NVSE_WheelSpdMean_kph]
  VVSE_RRwheelSpd_kph/1 -> [VVSE_RRwheelSpd_kph]
  Gain/1 -> Divide1/1
  [NVSE_WheelSpdMean_kph] -> Bias1/1
  [NVSE_WheelSpdMean_kph] -> Add/2
  Add1/1 -> Switch/2, Gain/1
  [NVSE_WheelSpdMean_kph] -> Add1/2
  [VVSE_RRwheelSpd_kph] -> Add1/1
  Bias1/1 -> Divide1/2
  Switch/1 -> VVSE_RRwheelSlip_rat/1  "VVSE_RRwheelSlip_rat"
  Divide/1 -> Switch/1
  Divide1/1 -> Switch/3

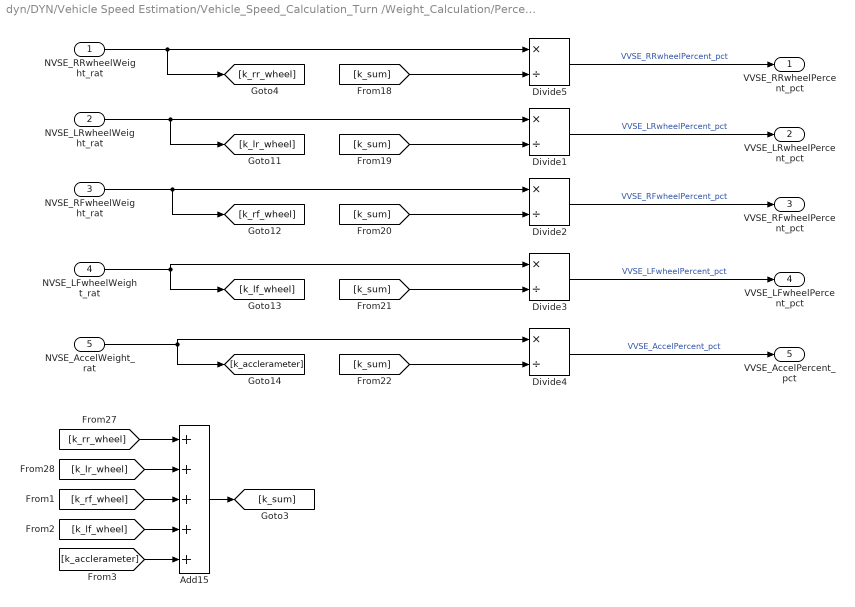
== system dyn/DYN/Vehicle Speed Estimation/Vehicle_Speed_Calculation_Turn /Weight_Calculation/Percentage ==
  NVSE_RRwheelWeight_rat : Inport
  NVSE_LRwheelWeight_rat : Inport  Port=2
  NVSE_RFwheelWeight_rat : Inport  Port=3
  NVSE_LFwheelWeight_rat : Inport  Port=4
  NVSE_AccelWeight_rat : Inport  Port=5
  Add15 : Sum  Inputs=+++++
  Divide{1..5} (5 alike) : Product  Inputs=*/
  VVSE_RRwheelPercent_pct : Outport
  VVSE_LRwheelPercent_pct : Outport  Port=2
  VVSE_RFwheelPercent_pct : Outport  Port=3
  VVSE_LFwheelPercent_pct : Outport  Port=4
  VVSE_AccelPercent_pct : Outport  Port=5
  wires:
  [k_sum] -> Divide1/2
  [k_sum] -> Divide3/2
  [k_sum] -> Divide2/2
  [k_sum] -> Divide4/2
  Add15/1 -> [k_sum]
  [k_acclerameter] -> Add15/5
  [k_lf_wheel] -> Add15/4
  [k_rf_wheel] -> Add15/3
  [k_lr_wheel] -> Add15/2
  [k_rr_wheel] -> Add15/1
  NVSE_RFwheelWeight_rat/1 -> [k_rf_wheel], Divide2/1
  Divide5/1 -> VVSE_RRwheelPercent_pct/1  "VVSE_RRwheelPercent_pct"
  Divide1/1 -> VVSE_LRwheelPercent_pct/1  "VVSE_LRwheelPercent_pct"
  Divide4/1 -> VVSE_AccelPercent_pct/1  "VVSE_AccelPercent_pct"
  [k_sum] -> Divide5/2
  NVSE_LRwheelWeight_rat/1 -> [k_lr_wheel], Divide1/1
  NVSE_RRwheelWeight_rat/1 -> [k_rr_wheel], Divide5/1
  Divide2/1 -> VVSE_RFwheelPercent_pct/1  "VVSE_RFwheelPercent_pct"
  Divide3/1 -> VVSE_LFwheelPercent_pct/1  "VVSE_LFwheelPercent_pct"
  NVSE_AccelWeight_rat/1 -> [k_acclerameter], Divide4/1
  NVSE_LFwheelWeight_rat/1 -> [k_lf_wheel], Divide3/1
